simulink model "sintonia_PID_exemplo"  (R2019b)
settings: Solver=ode45  StartTime=0.0  StopTime=7  RelTol=1e-3
settings Model: Creator=fernandopassold  LastModifiedBy=fernandopassold
settings DataIOCC: ReturnWorkspaceOutputs=off
settings DebuggingCC: ArithmeticOperatorsInVariantConditions=warning
settings SFSimCC: SimUseLocalCustomCode=off  CustomCodeUndefinedFunction=UseInterfaceOnly
settings RTWCC: RTWUseLocalCustomCode=off

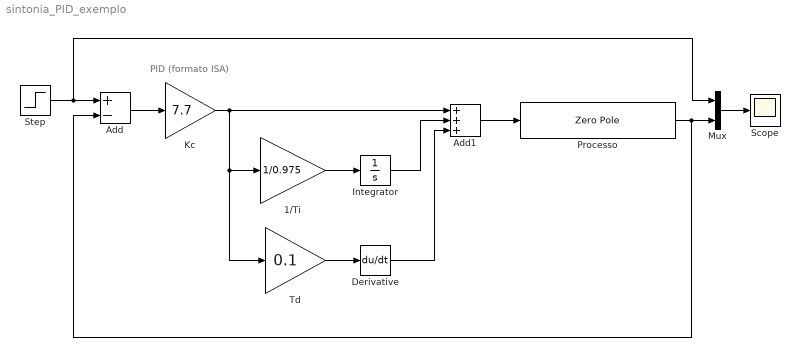
== system sintonia_PID_exemplo ==
  note: PID (formato ISA)
  1/Ti : Gain  Gain=1/0.975
  Add : Sum  Inputs=+-
  Add1 : Sum  Inputs=+++
  Derivative : Derivative
  Integrator : Integrator
  Kc : Gain  Gain=7.7
  Mux : Mux  Inputs=2
  Processo : ZeroPole  Zeros=[ ]  Poles=[-1 -4 -10]  Gain=[20]
  Scope : Scope
  Step : Step  SampleTime=0
  Td : Gain  Gain=0.1
  wires:
  Add/1 -> Kc/1
  Kc/1 -> Td/1, 1/Ti/1, Add1/1
  1/Ti/1 -> Integrator/1
  Td/1 -> Derivative/1
  Integrator/1 -> Add1/2
  Derivative/1 -> Add1/3
  Add1/1 -> Processo/1
  Processo/1 -> Add/2, Mux/2
  Step/1 -> Mux/1, Add/1
  Mux/1 -> Scope/1
